simulink model "Pedal_Interpretation_exe_gr"  (Simulink 7.0)
settings: Solver=ode4  StartTime=0.0  StopTime=88  FixedStep=0.01  RelTol=1e-3
InitFcn:
  | PedalInterp_para
values from neighbouring files (symbols this model uses):
  ped_min = 5    [PedalInterp_para.m]
  T_max_Brake = 4000    [PedalInterp_para.m]
  TI = 0    [PAS_callback.m]
undefined symbols (not defined in the file or in its folder): fzgbib, m_ab_100pro, m_ab_70pro, PedalInterpretation, v_bereich
libraries: simulink x320
(part 6 of 23)

== system Pedal_Interpretation_exe_gr/Test Specification for PI/SR-PI-02.1 Brake pedal interpretation/true/PS ==
  A TI1 : Inport  OutDataType=sfix(16)  OutScaling=2^0
  AND : Logic  Inputs=4  AllPortsSameDT=off  OutDataTypeMode=boolean
  Bus Creator : BusCreator  Inputs=3
  Data Type Conversion : DataTypeConversion  OutDataType=sfix(16)  OutScaling=2^0
  Data Type Conversion1 : DataTypeConversion  OutDataType=sfix(16)  OutScaling=2^0
  Data Type Conversion2 : DataTypeConversion  OutDataType=sfix(16)  OutScaling=2^0
  Max Delay A : Subsystem  TreatAsAtomicUnit=on  mask{Delay=0}
      mask prompts: Delay "Delay (in simulation steps) for the input signal:"
      mask init:
      | %set_param([gcb '/Discrete Transfer Fcn'],'Denominator',['[' num2str([1 zeros(1,str2double(get_param(gcb,'Delay')))]) ']']);
      mask CallbackString:
      | Delay = str2double(get_param(gcb,'Delay'));
      | if Delay < 0
      |     set_param(gcb,'Delay','0');
      |     error('Only non-negative delays are possible (causality).');
      |     set_param([gcb '/Delay'],'Value','0');
      | elseif Delay == 0
      |     set_param([gcb '/Delay'],'Value','0');
      | else
      |     set_param([gcb '/Integer Delay'],'NumDelays',num2str(Delay));
      |     set_param([gcb '/Delay'],'Value',num2str(Delay));
      | end
      mask Display: text(0.5,0.5,['z^{ ' num2str((-1)*str2double(get_param(gcb,'Delay'))) '}'],'texmode','on');
  Max Delay R : Subsystem  TreatAsAtomicUnit=on  mask{Delay=0}
      mask prompts: Delay "Delay (in simulation steps) for the input signal:"
      mask init:
      | %set_param([gcb '/Discrete Transfer Fcn'],'Denominator',['[' num2str([1 zeros(1,str2double(get_param(gcb,'Delay')))]) ']']);
      mask CallbackString:
      | Delay = str2double(get_param(gcb,'Delay'));
      | if Delay < 0
      |     set_param(gcb,'Delay','0');
      |     error('Only non-negative delays are possible (causality).');
      |     set_param([gcb '/Delay'],'Value','0');
      | elseif Delay == 0
      |     set_param([gcb '/Delay'],'Value','0');
      | else
      |     set_param([gcb '/Integer Delay'],'NumDelays',num2str(Delay));
      |     set_param([gcb '/Delay'],'Value',num2str(Delay));
      | end
      mask Display: text(0.5,0.5,['z^{ ' num2str((-1)*str2double(get_param(gcb,'Delay'))) '}'],'texmode','on');
  Max Delay T : Subsystem  TreatAsAtomicUnit=on  mask{Delay=0}
      mask prompts: Delay "Delay (in simulation steps) for the input signal:"
      mask init:
      | %set_param([gcb '/Discrete Transfer Fcn'],'Denominator',['[' num2str([1 zeros(1,str2double(get_param(gcb,'Delay')))]) ']']);
      mask CallbackString:
      | Delay = str2double(get_param(gcb,'Delay'));
      | if Delay < 0
      |     set_param(gcb,'Delay','0');
      |     error('Only non-negative delays are possible (causality).');
      |     set_param([gcb '/Delay'],'Value','0');
      | elseif Delay == 0
      |     set_param([gcb '/Delay'],'Value','0');
      | else
      |     set_param([gcb '/Integer Delay'],'NumDelays',num2str(Delay));
      |     set_param([gcb '/Delay'],'Value',num2str(Delay));
      | end
      mask Display: text(0.5,0.5,['z^{ ' num2str((-1)*str2double(get_param(gcb,'Delay'))) '}'],'texmode','on');
  OR - AND : Subsystem
  TDD : Subsystem
  TI : Subsystem
  TID : Subsystem
  Precond : Outport  OutDataType=sfix(16)  OutScaling=2^0
  wires:
  TDD/2(T) -> AND/4
  TID/2(T) -> Max Delay T/1(In1)
  TID/1(A) -> Max Delay A/1(In1)
  Bus Creator/1 -> Precond/1
  Data Type Conversion/1 -> Bus Creator/1  "A"
  Data Type Conversion1/1 -> Bus Creator/2  "T"
  TDD/1(A) -> AND/3
  Max Delay T/1(Out1) -> Data Type Conversion1/1
  Max Delay R/1(Out1) -> AND/1
  Max Delay A/1(Out1) -> Data Type Conversion/1
  AND/1 -> Data Type Conversion2/1
  OR - AND/2(AND) -> TID/2(R AND), Max Delay R/1(In1)
  OR - AND/1(OR) -> TID/1(R OR)
  TI/1(A) -> AND/2
  Data Type Conversion2/1 -> Bus Creator/3  "R"
  A TI1/1 -> TI/1(A1)

== system Pedal_Interpretation_exe_gr/Test Specification for PI/SR-PI-02.2 Acceleration pedal interpretation/T_des_Drive = const/Detect constant ==
  Signal : Inport  OutDataType=sfix(16)  OutScaling=2^0
  Clock : Clock
      settings: Decimation=10
  Constant1 : Constant  Value=0  OutDataTypeMode=boolean  OutDataType=sfix(16)  OutScaling=2^0
  Memory : Memory
  Relative tolerance : Subsystem
  Switch : Switch  Criteria=u2 > Threshold
  Constant : Outport  OutDataType=sfix(16)  OutScaling=2^0
  wires:
  Signal/1 -> Memory/1, Relative tolerance/1(sig)
  Memory/1 -> Relative tolerance/2(ref)
  Constant1/1 -> Switch/3
  Clock/1 -> Switch/2
  Relative tolerance/1(sig == ref) -> Switch/1
  Switch/1 -> Constant/1

== system Pedal_Interpretation_exe_gr/Test Specification for PI/SR-PI-02.2 Acceleration pedal interpretation/T_des_Drive = const/PAS ==
  Precond : Inport  OutDataType=sfix(16)  OutScaling=2^0
  V : Inport  Port=2  OutDataType=sfix(16)  OutScaling=2^0
  A delay : Subsystem  TreatAsAtomicUnit=on  mask{Delay=0}
      mask prompts: Delay "Delay (in simulation steps) for the input signal:"
      mask init:
      | %set_param([gcb '/Discrete Transfer Fcn'],'Denominator',['[' num2str([1 zeros(1,str2double(get_param(gcb,'Delay')))]) ']']);
      mask CallbackString:
      | Delay = str2double(get_param(gcb,'Delay'));
      | if Delay < 0
      |     set_param(gcb,'Delay','0');
      |     error('Only non-negative delays are possible (causality).');
      |     set_param([gcb '/Delay'],'Value','0');
      | elseif Delay == 0
      |     set_param([gcb '/Delay'],'Value','0');
      | else
      |     set_param([gcb '/Integer Delay'],'NumDelays',num2str(Delay));
      |     set_param([gcb '/Delay'],'Value',num2str(Delay));
      | end
      mask Display: text(0.5,0.5,['z^{ ' num2str((-1)*str2double(get_param(gcb,'Delay'))) '}'],'texmode','on');
  AND1 : Logic  AllPortsSameDT=off  OutDataTypeMode=boolean
  Bus Selector : BusSelector  OutputSignals=Local verdict
  Bus Selector1 : BusSelector  OutputSignals=Expected lower limit,Expected upper limit,Actual data
  Bus Selector2 : BusSelector  OutputSignals=R,T,A
  Bus Assignment : BusAssignment  AssignedSignals=Local verdict,Delay
  Bus Assignment1 : BusAssignment  AssignedSignals=Expected lower limit,Expected upper limit,Actual data
  Constant : Constant  Value=-1  OutDataType=sfix(16)  OutScaling=2^0
  Delay bus signals : Subsystem
  Ra delay : Subsystem  TreatAsAtomicUnit=on  mask{Delay=0}
      mask prompts: Delay "Delay (in simulation steps) for the input signal:"
      mask init:
      | %set_param([gcb '/Discrete Transfer Fcn'],'Denominator',['[' num2str([1 zeros(1,str2double(get_param(gcb,'Delay')))]) ']']);
      mask CallbackString:
      | Delay = str2double(get_param(gcb,'Delay'));
      | if Delay < 0
      |     set_param(gcb,'Delay','0');
      |     error('Only non-negative delays are possible (causality).');
      |     set_param([gcb '/Delay'],'Value','0');
      | elseif Delay == 0
      |     set_param([gcb '/Delay'],'Value','0');
      | else
      |     set_param([gcb '/Integer Delay'],'NumDelays',num2str(Delay));
      |     set_param([gcb '/Delay'],'Value',num2str(Delay));
      | end
      mask Display: text(0.5,0.5,['z^{ ' num2str((-1)*str2double(get_param(gcb,'Delay'))) '}'],'texmode','on');
  Rp delay : Subsystem  TreatAsAtomicUnit=on  mask{Delay=0}
      mask prompts: Delay "Delay (in simulation steps) for the input signal:"
      mask init:
      | %set_param([gcb '/Discrete Transfer Fcn'],'Denominator',['[' num2str([1 zeros(1,str2double(get_param(gcb,'Delay')))]) ']']);
      mask CallbackString:
      | Delay = str2double(get_param(gcb,'Delay'));
      | if Delay < 0
      |     set_param(gcb,'Delay','0');
      |     error('Only non-negative delays are possible (causality).');
      |     set_param([gcb '/Delay'],'Value','0');
      | elseif Delay == 0
      |     set_param([gcb '/Delay'],'Value','0');
      | else
      |     set_param([gcb '/Integer Delay'],'NumDelays',num2str(Delay));
      |     set_param([gcb '/Delay'],'Value',num2str(Delay));
      | end
      mask Display: text(0.5,0.5,['z^{ ' num2str((-1)*str2double(get_param(gcb,'Delay'))) '}'],'texmode','on');
  Ta delay : Subsystem  TreatAsAtomicUnit=on  mask{Delay=0}
      mask prompts: Delay "Delay (in simulation steps) for the input signal:"
      mask init:
      | %set_param([gcb '/Discrete Transfer Fcn'],'Denominator',['[' num2str([1 zeros(1,str2double(get_param(gcb,'Delay')))]) ']']);
      mask CallbackString:
      | Delay = str2double(get_param(gcb,'Delay'));
      | if Delay < 0
      |     set_param(gcb,'Delay','0');
      |     error('Only non-negative delays are possible (causality).');
      |     set_param([gcb '/Delay'],'Value','0');
      | elseif Delay == 0
      |     set_param([gcb '/Delay'],'Value','0');
      | else
      |     set_param([gcb '/Integer Delay'],'NumDelays',num2str(Delay));
      |     set_param([gcb '/Delay'],'Value',num2str(Delay));
      | end
      mask Display: text(0.5,0.5,['z^{ ' num2str((-1)*str2double(get_param(gcb,'Delay'))) '}'],'texmode','on');
  Tp delay : Subsystem  TreatAsAtomicUnit=on  mask{Delay=0}
      mask prompts: Delay "Delay (in simulation steps) for the input signal:"
      mask init:
      | %set_param([gcb '/Discrete Transfer Fcn'],'Denominator',['[' num2str([1 zeros(1,str2double(get_param(gcb,'Delay')))]) ']']);
      mask CallbackString:
      | Delay = str2double(get_param(gcb,'Delay'));
      | if Delay < 0
      |     set_param(gcb,'Delay','0');
      |     error('Only non-negative delays are possible (causality).');
      |     set_param([gcb '/Delay'],'Value','0');
      | elseif Delay == 0
      |     set_param([gcb '/Delay'],'Value','0');
      | else
      |     set_param([gcb '/Integer Delay'],'NumDelays',num2str(Delay));
      |     set_param([gcb '/Delay'],'Value',num2str(Delay));
      | end
      mask Display: text(0.5,0.5,['z^{ ' num2str((-1)*str2double(get_param(gcb,'Delay'))) '}'],'texmode','on');
  V delay : Subsystem  TreatAsAtomicUnit=on  mask{Delay=0}
      mask prompts: Delay "Delay (in simulation steps) for the input signal:"
      mask init:
      | %set_param([gcb '/Discrete Transfer Fcn'],'Denominator',['[' num2str([1 zeros(1,str2double(get_param(gcb,'Delay')))]) ']']);
      mask CallbackString:
      | Delay = str2double(get_param(gcb,'Delay'));
      | if Delay < 0
      |     set_param(gcb,'Delay','0');
      |     error('Only non-negative delays are possible (causality).');
      |     set_param([gcb '/Delay'],'Value','0');
      | elseif Delay == 0
      |     set_param([gcb '/Delay'],'Value','0');
      | else
      |     set_param([gcb '/Integer Delay'],'NumDelays',num2str(Delay));
      |     set_param([gcb '/Delay'],'Value',num2str(Delay));
      | end
      mask Display: text(0.5,0.5,['z^{ ' num2str((-1)*str2double(get_param(gcb,'Delay'))) '}'],'texmode','on');
  error : Subsystem
  none - pass - fail : Subsystem
  sw D : Switch  Criteria=u2 ~= 0
  sw V : Switch  Criteria=u2 ~= 0
  VF Info : Outport  OutDataType=sfix(16)  OutScaling=2^0
  wires:
  V/1 -> Bus Selector/1, Bus Selector1/1, Bus Assignment1/1
  error/1(Verror) -> sw V/2, sw D/2
  Constant/1 -> sw V/1
  none - pass - fail/1(Verdict) -> sw V/3
  none - pass - fail/2(MaxDelay) -> sw D/1
  none - pass - fail/3(Delay) -> sw D/3
  sw V/1 -> Bus Assignment/2
  sw D/1 -> Bus Assignment/3
  Bus Selector/1 -> V delay/1(In1), Ra delay/1(In1), Ta delay/1(In1)  "<Local verdict>"
  Bus Assignment/1 -> VF Info/1
  Bus Selector2/1 -> Rp delay/1(In1)  "<R>"
  Bus Selector2/2 -> Tp delay/1(In1)  "<T>"
  Bus Selector2/3 -> A delay/1(In1)  "<A>"
  Rp delay/1(Out1) -> error/1(Rp), none - pass - fail/1(Rp), AND1/1
  Tp delay/1(Out1) -> error/2(Tp), none - pass - fail/2(Tp)
  A delay/1(Out1) -> error/3(A), none - pass - fail/3(A)
  V delay/1(Out1) -> error/6(V), none - pass - fail/6(V)
  Ra delay/1(Out1) -> none - pass - fail/4(Ra), AND1/2, error/4(Ra)
  AND1/1 -> none - pass - fail/7(R AND)
  Precond/1 -> Bus Selector2/1
  Bus Selector1/1 -> Delay bus signals/1(ELLin)  "<Expected lower limit>"
  Bus Selector1/2 -> Delay bus signals/2(EULin)  "<Expected upper limit>"
  Bus Selector1/3 -> Delay bus signals/3(ADin)  "<Actual data>"
  Bus Assignment1/1 -> Bus Assignment/1
  Delay bus signals/1(ELLout) -> Bus Assignment1/2
  Delay bus signals/2(EULout) -> Bus Assignment1/3
  Delay bus signals/3(ADout) -> Bus Assignment1/4
  Ta delay/1(Out1) -> none - pass - fail/5(Ta), error/5(Ta)

== system Pedal_Interpretation_exe_gr/Test Specification for PI/SR-PI-02.2 Acceleration pedal interpretation/T_des_Drive = const/Range - Gap Relative tolerance Ass ==
  Signal : Inport  OutDataType=sfix(16)  OutScaling=2^0
  Reference : Inport  Port=2  OutDataType=sfix(16)  OutScaling=2^0
  Abs : Abs
  Abs1 : Abs
  Add : Sum  Inputs=+-  OutDataType=sfix(16)  OutScaling=2^-10
  Add1 : Sum  Inputs=+-  OutDataType=sfix(16)  OutScaling=2^-10
  Add2 : Sum  OutDataType=sfix(16)  OutScaling=2^-10
  Bus Creator : BusCreator  Inputs=5
  Data Type Conversion : DataTypeConversion  OutDataTypeMode=double  OutDataType=sfix(16)  OutScaling=2^0
  Data Type Conversion1 : DataTypeConversion  OutDataType=sfix(16)  OutScaling=2^0
  Data Type Conversion2 : DataTypeConversion  OutDataType=sfix(16)  OutScaling=2^0
  Data Type Conversion3 : DataTypeConversion  OutDataType=sfix(16)  OutScaling=2^0
  Delay : Constant  Value=0  OutDataType=sfix(16)  OutScaling=2^0
  Divide1 : Product  Inputs=**/  OutDataType=sfix(16)  OutScaling=2^-10
  Max : Constant  Value=100  OutDataType=sfix(16)  OutScaling=2^0
  Relational Operator : RelationalOperator  Operator=<=  LogicOutDataTypeMode=boolean
  Relative Tolerance : Constant  OutDataType=sfix(16)  OutScaling=2^0
  V : Outport  OutDataType=sfix(16)  OutScaling=2^0  InitialOutput=[2]
  wires:
  Data Type Conversion3/1 -> Bus Creator/4  "Actual data"
  Data Type Conversion2/1 -> Bus Creator/3  "Expected upper limit"
  Data Type Conversion1/1 -> Bus Creator/2  "Expected lower limit"
  Data Type Conversion/1 -> Bus Creator/1  "Local verdict"
  Bus Creator/1 -> V/1
  Add1/1 -> Data Type Conversion1/1
  Add2/1 -> Data Type Conversion2/1
  Delay/1 -> Bus Creator/5  "Delay"
  Abs1/1 -> Divide1/1
  Relational Operator/1 -> Data Type Conversion/1
  Relative Tolerance/1 -> Divide1/2
  Max/1 -> Divide1/3
  Divide1/1 -> Add2/1, Add1/2, Relational Operator/2
  Reference/1 -> Add1/1, Add2/2, Abs1/1, Add/2
  Signal/1 -> Data Type Conversion3/1, Add/1
  Add/1 -> Abs/1
  Abs/1 -> Relational Operator/1

== system Pedal_Interpretation_exe_gr/Test Specification for PI/SR-PI-02.2 Acceleration pedal interpretation/T_des_Drive decreases/Detect decrease ==
  Signal : Inport  OutDataType=sfix(16)  OutScaling=2^0
  Clock : Clock
      settings: Decimation=10
  Memory : Memory
  Relational Operator : RelationalOperator  Operator=<  LogicOutDataTypeMode=Specify via dialog
  Switch : Switch  Criteria=u2 > Threshold
  Decrease : Outport  OutDataType=sfix(16)  OutScaling=2^0
  wires:
  Switch/1 -> Relational Operator/2
  Memory/1 -> Switch/1
  Clock/1 -> Switch/2
  Relational Operator/1 -> Decrease/1
  Signal/1 -> Switch/3, Memory/1, Relational Operator/1

== system Pedal_Interpretation_exe_gr/Test Specification for PI/SR-PI-02.2 Acceleration pedal interpretation/T_des_Drive decreases/PAS ==
  Precond : Inport  OutDataType=sfix(16)  OutScaling=2^0
  V : Inport  Port=2  OutDataType=sfix(16)  OutScaling=2^0
  A delay : Subsystem  TreatAsAtomicUnit=on  mask{Delay=0}
      mask prompts: Delay "Delay (in simulation steps) for the input signal:"
      mask init:
      | %set_param([gcb '/Discrete Transfer Fcn'],'Denominator',['[' num2str([1 zeros(1,str2double(get_param(gcb,'Delay')))]) ']']);
      mask CallbackString:
      | Delay = str2double(get_param(gcb,'Delay'));
      | if Delay < 0
      |     set_param(gcb,'Delay','0');
      |     error('Only non-negative delays are possible (causality).');
      |     set_param([gcb '/Delay'],'Value','0');
      | elseif Delay == 0
      |     set_param([gcb '/Delay'],'Value','0');
      | else
      |     set_param([gcb '/Integer Delay'],'NumDelays',num2str(Delay));
      |     set_param([gcb '/Delay'],'Value',num2str(Delay));
      | end
      mask Display: text(0.5,0.5,['z^{ ' num2str((-1)*str2double(get_param(gcb,'Delay'))) '}'],'texmode','on');
  AND1 : Logic  AllPortsSameDT=off  OutDataTypeMode=boolean
  Bus Selector : BusSelector  OutputSignals=Local verdict
  Bus Selector1 : BusSelector  OutputSignals=Expected lower limit,Expected upper limit,Actual data
  Bus Selector2 : BusSelector  OutputSignals=R,T,A
  Bus Assignment : BusAssignment  AssignedSignals=Local verdict,Delay
  Bus Assignment1 : BusAssignment  AssignedSignals=Expected lower limit,Expected upper limit,Actual data
  Constant : Constant  Value=-1  OutDataType=sfix(16)  OutScaling=2^0
  Delay bus signals : Subsystem
  Ra delay : Subsystem  TreatAsAtomicUnit=on  mask{Delay=0}
      mask prompts: Delay "Delay (in simulation steps) for the input signal:"
      mask init:
      | %set_param([gcb '/Discrete Transfer Fcn'],'Denominator',['[' num2str([1 zeros(1,str2double(get_param(gcb,'Delay')))]) ']']);
      mask CallbackString:
      | Delay = str2double(get_param(gcb,'Delay'));
      | if Delay < 0
      |     set_param(gcb,'Delay','0');
      |     error('Only non-negative delays are possible (causality).');
      |     set_param([gcb '/Delay'],'Value','0');
      | elseif Delay == 0
      |     set_param([gcb '/Delay'],'Value','0');
      | else
      |     set_param([gcb '/Integer Delay'],'NumDelays',num2str(Delay));
      |     set_param([gcb '/Delay'],'Value',num2str(Delay));
      | end
      mask Display: text(0.5,0.5,['z^{ ' num2str((-1)*str2double(get_param(gcb,'Delay'))) '}'],'texmode','on');
  Rp delay : Subsystem  TreatAsAtomicUnit=on  mask{Delay=0}
      mask prompts: Delay "Delay (in simulation steps) for the input signal:"
      mask init:
      | %set_param([gcb '/Discrete Transfer Fcn'],'Denominator',['[' num2str([1 zeros(1,str2double(get_param(gcb,'Delay')))]) ']']);
      mask CallbackString:
      | Delay = str2double(get_param(gcb,'Delay'));
      | if Delay < 0
      |     set_param(gcb,'Delay','0');
      |     error('Only non-negative delays are possible (causality).');
      |     set_param([gcb '/Delay'],'Value','0');
      | elseif Delay == 0
      |     set_param([gcb '/Delay'],'Value','0');
      | else
      |     set_param([gcb '/Integer Delay'],'NumDelays',num2str(Delay));
      |     set_param([gcb '/Delay'],'Value',num2str(Delay));
      | end
      mask Display: text(0.5,0.5,['z^{ ' num2str((-1)*str2double(get_param(gcb,'Delay'))) '}'],'texmode','on');
  Ta delay : Subsystem  TreatAsAtomicUnit=on  mask{Delay=0}
      mask prompts: Delay "Delay (in simulation steps) for the input signal:"
      mask init:
      | %set_param([gcb '/Discrete Transfer Fcn'],'Denominator',['[' num2str([1 zeros(1,str2double(get_param(gcb,'Delay')))]) ']']);
      mask CallbackString:
      | Delay = str2double(get_param(gcb,'Delay'));
      | if Delay < 0
      |     set_param(gcb,'Delay','0');
      |     error('Only non-negative delays are possible (causality).');
      |     set_param([gcb '/Delay'],'Value','0');
      | elseif Delay == 0
      |     set_param([gcb '/Delay'],'Value','0');
      | else
      |     set_param([gcb '/Integer Delay'],'NumDelays',num2str(Delay));
      |     set_param([gcb '/Delay'],'Value',num2str(Delay));
      | end
      mask Display: text(0.5,0.5,['z^{ ' num2str((-1)*str2double(get_param(gcb,'Delay'))) '}'],'texmode','on');
  Tp delay : Subsystem  TreatAsAtomicUnit=on  mask{Delay=0}
      mask prompts: Delay "Delay (in simulation steps) for the input signal:"
      mask init:
      | %set_param([gcb '/Discrete Transfer Fcn'],'Denominator',['[' num2str([1 zeros(1,str2double(get_param(gcb,'Delay')))]) ']']);
      mask CallbackString:
      | Delay = str2double(get_param(gcb,'Delay'));
      | if Delay < 0
      |     set_param(gcb,'Delay','0');
      |     error('Only non-negative delays are possible (causality).');
      |     set_param([gcb '/Delay'],'Value','0');
      | elseif Delay == 0
      |     set_param([gcb '/Delay'],'Value','0');
      | else
      |     set_param([gcb '/Integer Delay'],'NumDelays',num2str(Delay));
      |     set_param([gcb '/Delay'],'Value',num2str(Delay));
      | end
      mask Display: text(0.5,0.5,['z^{ ' num2str((-1)*str2double(get_param(gcb,'Delay'))) '}'],'texmode','on');
  V delay : Subsystem  TreatAsAtomicUnit=on  mask{Delay=0}
      mask prompts: Delay "Delay (in simulation steps) for the input signal:"
      mask init:
      | %set_param([gcb '/Discrete Transfer Fcn'],'Denominator',['[' num2str([1 zeros(1,str2double(get_param(gcb,'Delay')))]) ']']);
      mask CallbackString:
      | Delay = str2double(get_param(gcb,'Delay'));
      | if Delay < 0
      |     set_param(gcb,'Delay','0');
      |     error('Only non-negative delays are possible (causality).');
      |     set_param([gcb '/Delay'],'Value','0');
      | elseif Delay == 0
      |     set_param([gcb '/Delay'],'Value','0');
      | else
      |     set_param([gcb '/Integer Delay'],'NumDelays',num2str(Delay));
      |     set_param([gcb '/Delay'],'Value',num2str(Delay));
      | end
      mask Display: text(0.5,0.5,['z^{ ' num2str((-1)*str2double(get_param(gcb,'Delay'))) '}'],'texmode','on');
  error : Subsystem
  none - pass - fail : Subsystem
  sw D : Switch  Criteria=u2 ~= 0
  sw V : Switch  Criteria=u2 ~= 0
  VF Info : Outport  OutDataType=sfix(16)  OutScaling=2^0
  wires:
  V/1 -> Bus Selector/1, Bus Selector1/1, Bus Assignment1/1
  error/1(Verror) -> sw V/2, sw D/2
  Constant/1 -> sw V/1
  none - pass - fail/1(Verdict) -> sw V/3
  none - pass - fail/2(MaxDelay) -> sw D/1
  none - pass - fail/3(Delay) -> sw D/3
  sw V/1 -> Bus Assignment/2
  sw D/1 -> Bus Assignment/3
  Bus Selector/1 -> V delay/1(In1), Ra delay/1(In1), Ta delay/1(In1)  "<Local verdict>"
  Bus Assignment/1 -> VF Info/1
  Bus Selector2/1 -> Rp delay/1(In1)  "<R>"
  Bus Selector2/2 -> Tp delay/1(In1)  "<T>"
  Bus Selector2/3 -> A delay/1(In1)  "<A>"
  Rp delay/1(Out1) -> error/1(Rp), none - pass - fail/1(Rp), AND1/1
  Tp delay/1(Out1) -> error/2(Tp), none - pass - fail/2(Tp)
  A delay/1(Out1) -> error/3(A), none - pass - fail/3(A)
  V delay/1(Out1) -> error/6(V), none - pass - fail/6(V)
  Ra delay/1(Out1) -> none - pass - fail/4(Ra), AND1/2, error/4(Ra)
  AND1/1 -> none - pass - fail/7(R AND)
  Precond/1 -> Bus Selector2/1
  Bus Selector1/1 -> Delay bus signals/1(ELLin)  "<Expected lower limit>"
  Bus Selector1/2 -> Delay bus signals/2(EULin)  "<Expected upper limit>"
  Bus Selector1/3 -> Delay bus signals/3(ADin)  "<Actual data>"
  Bus Assignment1/1 -> Bus Assignment/1
  Delay bus signals/1(ELLout) -> Bus Assignment1/2
  Delay bus signals/2(EULout) -> Bus Assignment1/3
  Delay bus signals/3(ADout) -> Bus Assignment1/4
  Ta delay/1(Out1) -> none - pass - fail/5(Ta), error/5(Ta)

== system Pedal_Interpretation_exe_gr/Test Specification for PI/SR-PI-02.2 Acceleration pedal interpretation/T_des_Drive decreases/Range - Gap Relative tolerance Ass ==
  Signal : Inport  OutDataType=sfix(16)  OutScaling=2^0
  Reference : Inport  Port=2  OutDataType=sfix(16)  OutScaling=2^0
  Abs : Abs
  Abs1 : Abs
  Add : Sum  Inputs=+-  OutDataType=sfix(16)  OutScaling=2^-10
  Add1 : Sum  Inputs=+-  OutDataType=sfix(16)  OutScaling=2^-10
  Add2 : Sum  OutDataType=sfix(16)  OutScaling=2^-10
  Bus Creator : BusCreator  Inputs=5
  Data Type Conversion : DataTypeConversion  OutDataTypeMode=double  OutDataType=sfix(16)  OutScaling=2^0
  Data Type Conversion1 : DataTypeConversion  OutDataType=sfix(16)  OutScaling=2^0
  Data Type Conversion2 : DataTypeConversion  OutDataType=sfix(16)  OutScaling=2^0
  Data Type Conversion3 : DataTypeConversion  OutDataType=sfix(16)  OutScaling=2^0
  Delay : Constant  Value=0  OutDataType=sfix(16)  OutScaling=2^0
  Divide1 : Product  Inputs=**/  OutDataType=sfix(16)  OutScaling=2^-10
  Max : Constant  Value=100  OutDataType=sfix(16)  OutScaling=2^0
  Relational Operator : RelationalOperator  Operator=<=  LogicOutDataTypeMode=boolean
  Relative Tolerance : Constant  OutDataType=sfix(16)  OutScaling=2^0
  V : Outport  OutDataType=sfix(16)  OutScaling=2^0  InitialOutput=[2]
  wires:
  Data Type Conversion3/1 -> Bus Creator/4  "Actual data"
  Data Type Conversion2/1 -> Bus Creator/3  "Expected upper limit"
  Data Type Conversion1/1 -> Bus Creator/2  "Expected lower limit"
  Data Type Conversion/1 -> Bus Creator/1  "Local verdict"
  Bus Creator/1 -> V/1
  Add1/1 -> Data Type Conversion1/1
  Add2/1 -> Data Type Conversion2/1
  Delay/1 -> Bus Creator/5  "Delay"
  Abs1/1 -> Divide1/1
  Relational Operator/1 -> Data Type Conversion/1
  Relative Tolerance/1 -> Divide1/2
  Max/1 -> Divide1/3
  Divide1/1 -> Add2/1, Add1/2, Relational Operator/2
  Reference/1 -> Add1/1, Add2/2, Abs1/1, Add/2
  Signal/1 -> Data Type Conversion3/1, Add/1
  Add/1 -> Abs/1
  Abs/1 -> Relational Operator/1

== system Pedal_Interpretation_exe_gr/Test Specification for PI/SR-PI-02.2 Acceleration pedal interpretation/T_des_Drive decreases /Detect decrease ==
  Signal : Inport  OutDataType=sfix(16)  OutScaling=2^0
  Clock : Clock
      settings: Decimation=10
  Memory : Memory
  Relational Operator : RelationalOperator  Operator=<  LogicOutDataTypeMode=Specify via dialog
  Switch : Switch  Criteria=u2 > Threshold
  Decrease : Outport  OutDataType=sfix(16)  OutScaling=2^0
  wires:
  Switch/1 -> Relational Operator/2
  Memory/1 -> Switch/1
  Clock/1 -> Switch/2
  Relational Operator/1 -> Decrease/1
  Signal/1 -> Switch/3, Memory/1, Relational Operator/1

== system Pedal_Interpretation_exe_gr/Test Specification for PI/SR-PI-02.2 Acceleration pedal interpretation/T_des_Drive decreases /PAS ==
  Precond : Inport  OutDataType=sfix(16)  OutScaling=2^0
  V : Inport  Port=2  OutDataType=sfix(16)  OutScaling=2^0
  A delay : Subsystem  TreatAsAtomicUnit=on  mask{Delay=0}
      mask prompts: Delay "Delay (in simulation steps) for the input signal:"
      mask init:
      | %set_param([gcb '/Discrete Transfer Fcn'],'Denominator',['[' num2str([1 zeros(1,str2double(get_param(gcb,'Delay')))]) ']']);
      mask CallbackString:
      | Delay = str2double(get_param(gcb,'Delay'));
      | if Delay < 0
      |     set_param(gcb,'Delay','0');
      |     error('Only non-negative delays are possible (causality).');
      |     set_param([gcb '/Delay'],'Value','0');
      | elseif Delay == 0
      |     set_param([gcb '/Delay'],'Value','0');
      | else
      |     set_param([gcb '/Integer Delay'],'NumDelays',num2str(Delay));
      |     set_param([gcb '/Delay'],'Value',num2str(Delay));
      | end
      mask Display: text(0.5,0.5,['z^{ ' num2str((-1)*str2double(get_param(gcb,'Delay'))) '}'],'texmode','on');
  AND1 : Logic  AllPortsSameDT=off  OutDataTypeMode=boolean
  Bus Selector : BusSelector  OutputSignals=Local verdict
  Bus Selector1 : BusSelector  OutputSignals=Expected lower limit,Expected upper limit,Actual data
  Bus Selector2 : BusSelector  OutputSignals=R,T,A
  Bus Assignment : BusAssignment  AssignedSignals=Local verdict,Delay
  Bus Assignment1 : BusAssignment  AssignedSignals=Expected lower limit,Expected upper limit,Actual data
  Constant : Constant  Value=-1  OutDataType=sfix(16)  OutScaling=2^0
  Delay bus signals : Subsystem
  Ra delay : Subsystem  TreatAsAtomicUnit=on  mask{Delay=0}
      mask prompts: Delay "Delay (in simulation steps) for the input signal:"
      mask init:
      | %set_param([gcb '/Discrete Transfer Fcn'],'Denominator',['[' num2str([1 zeros(1,str2double(get_param(gcb,'Delay')))]) ']']);
      mask CallbackString:
      | Delay = str2double(get_param(gcb,'Delay'));
      | if Delay < 0
      |     set_param(gcb,'Delay','0');
      |     error('Only non-negative delays are possible (causality).');
      |     set_param([gcb '/Delay'],'Value','0');
      | elseif Delay == 0
      |     set_param([gcb '/Delay'],'Value','0');
      | else
      |     set_param([gcb '/Integer Delay'],'NumDelays',num2str(Delay));
      |     set_param([gcb '/Delay'],'Value',num2str(Delay));
      | end
      mask Display: text(0.5,0.5,['z^{ ' num2str((-1)*str2double(get_param(gcb,'Delay'))) '}'],'texmode','on');
  Rp delay : Subsystem  TreatAsAtomicUnit=on  mask{Delay=0}
      mask prompts: Delay "Delay (in simulation steps) for the input signal:"
      mask init:
      | %set_param([gcb '/Discrete Transfer Fcn'],'Denominator',['[' num2str([1 zeros(1,str2double(get_param(gcb,'Delay')))]) ']']);
      mask CallbackString:
      | Delay = str2double(get_param(gcb,'Delay'));
      | if Delay < 0
      |     set_param(gcb,'Delay','0');
      |     error('Only non-negative delays are possible (causality).');
      |     set_param([gcb '/Delay'],'Value','0');
      | elseif Delay == 0
      |     set_param([gcb '/Delay'],'Value','0');
      | else
      |     set_param([gcb '/Integer Delay'],'NumDelays',num2str(Delay));
      |     set_param([gcb '/Delay'],'Value',num2str(Delay));
      | end
      mask Display: text(0.5,0.5,['z^{ ' num2str((-1)*str2double(get_param(gcb,'Delay'))) '}'],'texmode','on');
  Ta delay : Subsystem  TreatAsAtomicUnit=on  mask{Delay=0}
      mask prompts: Delay "Delay (in simulation steps) for the input signal:"
      mask init:
      | %set_param([gcb '/Discrete Transfer Fcn'],'Denominator',['[' num2str([1 zeros(1,str2double(get_param(gcb,'Delay')))]) ']']);
      mask CallbackString:
      | Delay = str2double(get_param(gcb,'Delay'));
      | if Delay < 0
      |     set_param(gcb,'Delay','0');
      |     error('Only non-negative delays are possible (causality).');
      |     set_param([gcb '/Delay'],'Value','0');
      | elseif Delay == 0
      |     set_param([gcb '/Delay'],'Value','0');
      | else
      |     set_param([gcb '/Integer Delay'],'NumDelays',num2str(Delay));
      |     set_param([gcb '/Delay'],'Value',num2str(Delay));
      | end
      mask Display: text(0.5,0.5,['z^{ ' num2str((-1)*str2double(get_param(gcb,'Delay'))) '}'],'texmode','on');
  Tp delay : Subsystem  TreatAsAtomicUnit=on  mask{Delay=0}
      mask prompts: Delay "Delay (in simulation steps) for the input signal:"
      mask init:
      | %set_param([gcb '/Discrete Transfer Fcn'],'Denominator',['[' num2str([1 zeros(1,str2double(get_param(gcb,'Delay')))]) ']']);
      mask CallbackString:
      | Delay = str2double(get_param(gcb,'Delay'));
      | if Delay < 0
      |     set_param(gcb,'Delay','0');
      |     error('Only non-negative delays are possible (causality).');
      |     set_param([gcb '/Delay'],'Value','0');
      | elseif Delay == 0
      |     set_param([gcb '/Delay'],'Value','0');
      | else
      |     set_param([gcb '/Integer Delay'],'NumDelays',num2str(Delay));
      |     set_param([gcb '/Delay'],'Value',num2str(Delay));
      | end
      mask Display: text(0.5,0.5,['z^{ ' num2str((-1)*str2double(get_param(gcb,'Delay'))) '}'],'texmode','on');
  V delay : Subsystem  TreatAsAtomicUnit=on  mask{Delay=0}
      mask prompts: Delay "Delay (in simulation steps) for the input signal:"
      mask init:
      | %set_param([gcb '/Discrete Transfer Fcn'],'Denominator',['[' num2str([1 zeros(1,str2double(get_param(gcb,'Delay')))]) ']']);
      mask CallbackString:
      | Delay = str2double(get_param(gcb,'Delay'));
      | if Delay < 0
      |     set_param(gcb,'Delay','0');
      |     error('Only non-negative delays are possible (causality).');
      |     set_param([gcb '/Delay'],'Value','0');
      | elseif Delay == 0
      |     set_param([gcb '/Delay'],'Value','0');
      | else
      |     set_param([gcb '/Integer Delay'],'NumDelays',num2str(Delay));
      |     set_param([gcb '/Delay'],'Value',num2str(Delay));
      | end
      mask Display: text(0.5,0.5,['z^{ ' num2str((-1)*str2double(get_param(gcb,'Delay'))) '}'],'texmode','on');
  error : Subsystem
  none - pass - fail : Subsystem
  sw D : Switch  Criteria=u2 ~= 0
  sw V : Switch  Criteria=u2 ~= 0
  VF Info : Outport  OutDataType=sfix(16)  OutScaling=2^0
  wires:
  V/1 -> Bus Selector/1, Bus Selector1/1, Bus Assignment1/1
  error/1(Verror) -> sw V/2, sw D/2
  Constant/1 -> sw V/1
  none - pass - fail/1(Verdict) -> sw V/3
  none - pass - fail/2(MaxDelay) -> sw D/1
  none - pass - fail/3(Delay) -> sw D/3
  sw V/1 -> Bus Assignment/2
  sw D/1 -> Bus Assignment/3
  Bus Selector/1 -> V delay/1(In1), Ra delay/1(In1), Ta delay/1(In1)  "<Local verdict>"
  Bus Assignment/1 -> VF Info/1
  Bus Selector2/1 -> Rp delay/1(In1)  "<R>"
  Bus Selector2/2 -> Tp delay/1(In1)  "<T>"
  Bus Selector2/3 -> A delay/1(In1)  "<A>"
  Rp delay/1(Out1) -> error/1(Rp), none - pass - fail/1(Rp), AND1/1
  Tp delay/1(Out1) -> error/2(Tp), none - pass - fail/2(Tp)
  A delay/1(Out1) -> error/3(A), none - pass - fail/3(A)
  V delay/1(Out1) -> error/6(V), none - pass - fail/6(V)
  Ra delay/1(Out1) -> none - pass - fail/4(Ra), AND1/2, error/4(Ra)
  AND1/1 -> none - pass - fail/7(R AND)
  Precond/1 -> Bus Selector2/1
  Bus Selector1/1 -> Delay bus signals/1(ELLin)  "<Expected lower limit>"
  Bus Selector1/2 -> Delay bus signals/2(EULin)  "<Expected upper limit>"
  Bus Selector1/3 -> Delay bus signals/3(ADin)  "<Actual data>"
  Bus Assignment1/1 -> Bus Assignment/1
  Delay bus signals/1(ELLout) -> Bus Assignment1/2
  Delay bus signals/2(EULout) -> Bus Assignment1/3
  Delay bus signals/3(ADout) -> Bus Assignment1/4
  Ta delay/1(Out1) -> none - pass - fail/5(Ta), error/5(Ta)

== system Pedal_Interpretation_exe_gr/Test Specification for PI/SR-PI-02.2 Acceleration pedal interpretation/T_des_Drive decreases /Range - Gap Relative tolerance Ass ==
  Signal : Inport  OutDataType=sfix(16)  OutScaling=2^0
  Reference : Inport  Port=2  OutDataType=sfix(16)  OutScaling=2^0
  Abs : Abs
  Abs1 : Abs
  Add : Sum  Inputs=+-  OutDataType=sfix(16)  OutScaling=2^-10
  Add1 : Sum  Inputs=+-  OutDataType=sfix(16)  OutScaling=2^-10
  Add2 : Sum  OutDataType=sfix(16)  OutScaling=2^-10
  Bus Creator : BusCreator  Inputs=5
  Data Type Conversion : DataTypeConversion  OutDataTypeMode=double  OutDataType=sfix(16)  OutScaling=2^0
  Data Type Conversion1 : DataTypeConversion  OutDataType=sfix(16)  OutScaling=2^0
  Data Type Conversion2 : DataTypeConversion  OutDataType=sfix(16)  OutScaling=2^0
  Data Type Conversion3 : DataTypeConversion  OutDataType=sfix(16)  OutScaling=2^0
  Delay : Constant  Value=0  OutDataType=sfix(16)  OutScaling=2^0
  Divide1 : Product  Inputs=**/  OutDataType=sfix(16)  OutScaling=2^-10
  Max : Constant  Value=100  OutDataType=sfix(16)  OutScaling=2^0
  Relational Operator : RelationalOperator  Operator=<=  LogicOutDataTypeMode=boolean
  Relative Tolerance : Constant  OutDataType=sfix(16)  OutScaling=2^0
  V : Outport  OutDataType=sfix(16)  OutScaling=2^0  InitialOutput=[2]
  wires:
  Data Type Conversion3/1 -> Bus Creator/4  "Actual data"
  Data Type Conversion2/1 -> Bus Creator/3  "Expected upper limit"
  Data Type Conversion1/1 -> Bus Creator/2  "Expected lower limit"
  Data Type Conversion/1 -> Bus Creator/1  "Local verdict"
  Bus Creator/1 -> V/1
  Add1/1 -> Data Type Conversion1/1
  Add2/1 -> Data Type Conversion2/1
  Delay/1 -> Bus Creator/5  "Delay"
  Abs1/1 -> Divide1/1
  Relational Operator/1 -> Data Type Conversion/1
  Relative Tolerance/1 -> Divide1/2
  Max/1 -> Divide1/3
  Divide1/1 -> Add2/1, Add1/2, Relational Operator/2
  Reference/1 -> Add1/1, Add2/2, Abs1/1, Add/2
  Signal/1 -> Data Type Conversion3/1, Add/1
  Add/1 -> Abs/1
  Abs/1 -> Relational Operator/1

== system Pedal_Interpretation_exe_gr/Test Specification for PI/SR-PI-02.2 Acceleration pedal interpretation/T_des_Drive does not increase/Detect 'does not increase' ==
  Signal : Inport  OutDataType=sfix(16)  OutScaling=2^0
  Clock : Clock
      settings: Decimation=10
  Memory : Memory
  Relational Operator : RelationalOperator  Operator=<=  LogicOutDataTypeMode=Specify via dialog
  Switch : Switch  Criteria=u2 > Threshold
  Decrease : Outport  OutDataType=sfix(16)  OutScaling=2^0
  wires:
  Switch/1 -> Relational Operator/2
  Memory/1 -> Switch/1
  Clock/1 -> Switch/2
  Relational Operator/1 -> Decrease/1
  Signal/1 -> Switch/3, Memory/1, Relational Operator/1

== system Pedal_Interpretation_exe_gr/Test Specification for PI/SR-PI-02.2 Acceleration pedal interpretation/T_des_Drive does not increase/PAS ==
  Precond : Inport  OutDataType=sfix(16)  OutScaling=2^0
  V : Inport  Port=2  OutDataType=sfix(16)  OutScaling=2^0
  A delay : Subsystem  TreatAsAtomicUnit=on  mask{Delay=0}
      mask prompts: Delay "Delay (in simulation steps) for the input signal:"
      mask init:
      | %set_param([gcb '/Discrete Transfer Fcn'],'Denominator',['[' num2str([1 zeros(1,str2double(get_param(gcb,'Delay')))]) ']']);
      mask CallbackString:
      | Delay = str2double(get_param(gcb,'Delay'));
      | if Delay < 0
      |     set_param(gcb,'Delay','0');
      |     error('Only non-negative delays are possible (causality).');
      |     set_param([gcb '/Delay'],'Value','0');
      | elseif Delay == 0
      |     set_param([gcb '/Delay'],'Value','0');
      | else
      |     set_param([gcb '/Integer Delay'],'NumDelays',num2str(Delay));
      |     set_param([gcb '/Delay'],'Value',num2str(Delay));
      | end
      mask Display: text(0.5,0.5,['z^{ ' num2str((-1)*str2double(get_param(gcb,'Delay'))) '}'],'texmode','on');
  AND1 : Logic  AllPortsSameDT=off  OutDataTypeMode=boolean
  Bus Selector : BusSelector  OutputSignals=Local verdict
  Bus Selector1 : BusSelector  OutputSignals=Expected lower limit,Expected upper limit,Actual data
  Bus Selector2 : BusSelector  OutputSignals=R,T,A
  Bus Assignment : BusAssignment  AssignedSignals=Local verdict,Delay
  Bus Assignment1 : BusAssignment  AssignedSignals=Expected lower limit,Expected upper limit,Actual data
  Constant : Constant  Value=-1  OutDataType=sfix(16)  OutScaling=2^0
  Delay bus signals : Subsystem
  Ra delay : Subsystem  TreatAsAtomicUnit=on  mask{Delay=0}
      mask prompts: Delay "Delay (in simulation steps) for the input signal:"
      mask init:
      | %set_param([gcb '/Discrete Transfer Fcn'],'Denominator',['[' num2str([1 zeros(1,str2double(get_param(gcb,'Delay')))]) ']']);
      mask CallbackString:
      | Delay = str2double(get_param(gcb,'Delay'));
      | if Delay < 0
      |     set_param(gcb,'Delay','0');
      |     error('Only non-negative delays are possible (causality).');
      |     set_param([gcb '/Delay'],'Value','0');
      | elseif Delay == 0
      |     set_param([gcb '/Delay'],'Value','0');
      | else
      |     set_param([gcb '/Integer Delay'],'NumDelays',num2str(Delay));
      |     set_param([gcb '/Delay'],'Value',num2str(Delay));
      | end
      mask Display: text(0.5,0.5,['z^{ ' num2str((-1)*str2double(get_param(gcb,'Delay'))) '}'],'texmode','on');
  Rp delay : Subsystem  TreatAsAtomicUnit=on  mask{Delay=0}
      mask prompts: Delay "Delay (in simulation steps) for the input signal:"
      mask init:
      | %set_param([gcb '/Discrete Transfer Fcn'],'Denominator',['[' num2str([1 zeros(1,str2double(get_param(gcb,'Delay')))]) ']']);
      mask CallbackString:
      | Delay = str2double(get_param(gcb,'Delay'));
      | if Delay < 0
      |     set_param(gcb,'Delay','0');
      |     error('Only non-negative delays are possible (causality).');
      |     set_param([gcb '/Delay'],'Value','0');
      | elseif Delay == 0
      |     set_param([gcb '/Delay'],'Value','0');
      | else
      |     set_param([gcb '/Integer Delay'],'NumDelays',num2str(Delay));
      |     set_param([gcb '/Delay'],'Value',num2str(Delay));
      | end
      mask Display: text(0.5,0.5,['z^{ ' num2str((-1)*str2double(get_param(gcb,'Delay'))) '}'],'texmode','on');
  Ta delay : Subsystem  TreatAsAtomicUnit=on  mask{Delay=0}
      mask prompts: Delay "Delay (in simulation steps) for the input signal:"
      mask init:
      | %set_param([gcb '/Discrete Transfer Fcn'],'Denominator',['[' num2str([1 zeros(1,str2double(get_param(gcb,'Delay')))]) ']']);
      mask CallbackString:
      | Delay = str2double(get_param(gcb,'Delay'));
      | if Delay < 0
      |     set_param(gcb,'Delay','0');
      |     error('Only non-negative delays are possible (causality).');
      |     set_param([gcb '/Delay'],'Value','0');
      | elseif Delay == 0
      |     set_param([gcb '/Delay'],'Value','0');
      | else
      |     set_param([gcb '/Integer Delay'],'NumDelays',num2str(Delay));
      |     set_param([gcb '/Delay'],'Value',num2str(Delay));
      | end
      mask Display: text(0.5,0.5,['z^{ ' num2str((-1)*str2double(get_param(gcb,'Delay'))) '}'],'texmode','on');
  Tp delay : Subsystem  TreatAsAtomicUnit=on  mask{Delay=0}
      mask prompts: Delay "Delay (in simulation steps) for the input signal:"
      mask init:
      | %set_param([gcb '/Discrete Transfer Fcn'],'Denominator',['[' num2str([1 zeros(1,str2double(get_param(gcb,'Delay')))]) ']']);
      mask CallbackString:
      | Delay = str2double(get_param(gcb,'Delay'));
      | if Delay < 0
      |     set_param(gcb,'Delay','0');
      |     error('Only non-negative delays are possible (causality).');
      |     set_param([gcb '/Delay'],'Value','0');
      | elseif Delay == 0
      |     set_param([gcb '/Delay'],'Value','0');
      | else
      |     set_param([gcb '/Integer Delay'],'NumDelays',num2str(Delay));
      |     set_param([gcb '/Delay'],'Value',num2str(Delay));
      | end
      mask Display: text(0.5,0.5,['z^{ ' num2str((-1)*str2double(get_param(gcb,'Delay'))) '}'],'texmode','on');
  V delay : Subsystem  TreatAsAtomicUnit=on  mask{Delay=0}
      mask prompts: Delay "Delay (in simulation steps) for the input signal:"
      mask init:
      | %set_param([gcb '/Discrete Transfer Fcn'],'Denominator',['[' num2str([1 zeros(1,str2double(get_param(gcb,'Delay')))]) ']']);
      mask CallbackString:
      | Delay = str2double(get_param(gcb,'Delay'));
      | if Delay < 0
      |     set_param(gcb,'Delay','0');
      |     error('Only non-negative delays are possible (causality).');
      |     set_param([gcb '/Delay'],'Value','0');
      | elseif Delay == 0
      |     set_param([gcb '/Delay'],'Value','0');
      | else
      |     set_param([gcb '/Integer Delay'],'NumDelays',num2str(Delay));
      |     set_param([gcb '/Delay'],'Value',num2str(Delay));
      | end
      mask Display: text(0.5,0.5,['z^{ ' num2str((-1)*str2double(get_param(gcb,'Delay'))) '}'],'texmode','on');
  error : Subsystem
  none - pass - fail : Subsystem
  sw D : Switch  Criteria=u2 ~= 0
  sw V : Switch  Criteria=u2 ~= 0
  VF Info : Outport  OutDataType=sfix(16)  OutScaling=2^0
  wires:
  V/1 -> Bus Selector/1, Bus Selector1/1, Bus Assignment1/1
  error/1(Verror) -> sw V/2, sw D/2
  Constant/1 -> sw V/1
  none - pass - fail/1(Verdict) -> sw V/3
  none - pass - fail/2(MaxDelay) -> sw D/1
  none - pass - fail/3(Delay) -> sw D/3
  sw V/1 -> Bus Assignment/2
  sw D/1 -> Bus Assignment/3
  Bus Selector/1 -> V delay/1(In1), Ra delay/1(In1), Ta delay/1(In1)  "<Local verdict>"
  Bus Assignment/1 -> VF Info/1
  Bus Selector2/1 -> Rp delay/1(In1)  "<R>"
  Bus Selector2/2 -> Tp delay/1(In1)  "<T>"
  Bus Selector2/3 -> A delay/1(In1)  "<A>"
  Rp delay/1(Out1) -> error/1(Rp), none - pass - fail/1(Rp), AND1/1
  Tp delay/1(Out1) -> error/2(Tp), none - pass - fail/2(Tp)
  A delay/1(Out1) -> error/3(A), none - pass - fail/3(A)
  V delay/1(Out1) -> error/6(V), none - pass - fail/6(V)
  Ra delay/1(Out1) -> none - pass - fail/4(Ra), AND1/2, error/4(Ra)
  AND1/1 -> none - pass - fail/7(R AND)
  Precond/1 -> Bus Selector2/1
  Bus Selector1/1 -> Delay bus signals/1(ELLin)  "<Expected lower limit>"
  Bus Selector1/2 -> Delay bus signals/2(EULin)  "<Expected upper limit>"
  Bus Selector1/3 -> Delay bus signals/3(ADin)  "<Actual data>"
  Bus Assignment1/1 -> Bus Assignment/1
  Delay bus signals/1(ELLout) -> Bus Assignment1/2
  Delay bus signals/2(EULout) -> Bus Assignment1/3
  Delay bus signals/3(ADout) -> Bus Assignment1/4
  Ta delay/1(Out1) -> none - pass - fail/5(Ta), error/5(Ta)

== system Pedal_Interpretation_exe_gr/Test Specification for PI/SR-PI-02.2 Acceleration pedal interpretation/T_des_Drive does not increase/Range - Gap Relative tolerance Ass ==
  Signal : Inport  OutDataType=sfix(16)  OutScaling=2^0
  Reference : Inport  Port=2  OutDataType=sfix(16)  OutScaling=2^0
  Abs : Abs
  Abs1 : Abs
  Add : Sum  Inputs=+-  OutDataType=sfix(16)  OutScaling=2^-10
  Add1 : Sum  Inputs=+-  OutDataType=sfix(16)  OutScaling=2^-10
  Add2 : Sum  OutDataType=sfix(16)  OutScaling=2^-10
  Bus Creator : BusCreator  Inputs=5
  Data Type Conversion : DataTypeConversion  OutDataTypeMode=double  OutDataType=sfix(16)  OutScaling=2^0
  Data Type Conversion1 : DataTypeConversion  OutDataType=sfix(16)  OutScaling=2^0
  Data Type Conversion2 : DataTypeConversion  OutDataType=sfix(16)  OutScaling=2^0
  Data Type Conversion3 : DataTypeConversion  OutDataType=sfix(16)  OutScaling=2^0
  Delay : Constant  Value=0  OutDataType=sfix(16)  OutScaling=2^0
  Divide1 : Product  Inputs=**/  OutDataType=sfix(16)  OutScaling=2^-10
  Max : Constant  Value=100  OutDataType=sfix(16)  OutScaling=2^0
  Relational Operator : RelationalOperator  Operator=<=  LogicOutDataTypeMode=boolean
  Relative Tolerance : Constant  OutDataType=sfix(16)  OutScaling=2^0
  V : Outport  OutDataType=sfix(16)  OutScaling=2^0  InitialOutput=[2]
  wires:
  Data Type Conversion3/1 -> Bus Creator/4  "Actual data"
  Data Type Conversion2/1 -> Bus Creator/3  "Expected upper limit"
  Data Type Conversion1/1 -> Bus Creator/2  "Expected lower limit"
  Data Type Conversion/1 -> Bus Creator/1  "Local verdict"
  Bus Creator/1 -> V/1
  Add1/1 -> Data Type Conversion1/1
  Add2/1 -> Data Type Conversion2/1
  Delay/1 -> Bus Creator/5  "Delay"
  Abs1/1 -> Divide1/1
  Relational Operator/1 -> Data Type Conversion/1
  Relative Tolerance/1 -> Divide1/2
  Max/1 -> Divide1/3
  Divide1/1 -> Add2/1, Add1/2, Relational Operator/2
  Reference/1 -> Add1/1, Add2/2, Abs1/1, Add/2
  Signal/1 -> Data Type Conversion3/1, Add/1
  Add/1 -> Abs/1
  Abs/1 -> Relational Operator/1

== system Pedal_Interpretation_exe_gr/Test Specification for PI/SR-PI-02.2 Acceleration pedal interpretation/T_des_Drive increases/   ==
  Signal : Inport  OutDataType=sfix(16)  OutScaling=2^0
  Reference : Inport  Port=2  OutDataType=sfix(16)  OutScaling=2^0
  Abs : Abs
  Abs1 : Abs
  Add : Sum  Inputs=+-  OutDataType=sfix(16)  OutScaling=2^-10
  Add1 : Sum  Inputs=+-  OutDataType=sfix(16)  OutScaling=2^-10
  Add2 : Sum  OutDataType=sfix(16)  OutScaling=2^-10
  Bus Creator : BusCreator  Inputs=5
  Data Type Conversion : DataTypeConversion  OutDataTypeMode=double  OutDataType=sfix(16)  OutScaling=2^0
  Data Type Conversion1 : DataTypeConversion  OutDataType=sfix(16)  OutScaling=2^0
  Data Type Conversion2 : DataTypeConversion  OutDataType=sfix(16)  OutScaling=2^0
  Data Type Conversion3 : DataTypeConversion  OutDataType=sfix(16)  OutScaling=2^0
  Delay : Constant  Value=0  OutDataType=sfix(16)  OutScaling=2^0
  Divide1 : Product  Inputs=**/  OutDataType=sfix(16)  OutScaling=2^-10
  Max : Constant  Value=100  OutDataType=sfix(16)  OutScaling=2^0
  Relational Operator : RelationalOperator  Operator=<=  LogicOutDataTypeMode=boolean
  Relative Tolerance : Constant  OutDataType=sfix(16)  OutScaling=2^0
  V : Outport  OutDataType=sfix(16)  OutScaling=2^0  InitialOutput=[2]
  wires:
  Data Type Conversion3/1 -> Bus Creator/4  "Actual data"
  Data Type Conversion2/1 -> Bus Creator/3  "Expected upper limit"
  Data Type Conversion1/1 -> Bus Creator/2  "Expected lower limit"
  Data Type Conversion/1 -> Bus Creator/1  "Local verdict"
  Bus Creator/1 -> V/1
  Add1/1 -> Data Type Conversion1/1
  Add2/1 -> Data Type Conversion2/1
  Delay/1 -> Bus Creator/5  "Delay"
  Abs1/1 -> Divide1/1
  Relational Operator/1 -> Data Type Conversion/1
  Relative Tolerance/1 -> Divide1/2
  Max/1 -> Divide1/3
  Divide1/1 -> Add2/1, Add1/2, Relational Operator/2
  Reference/1 -> Add1/1, Add2/2, Abs1/1, Add/2
  Signal/1 -> Data Type Conversion3/1, Add/1
  Add/1 -> Abs/1
  Abs/1 -> Relational Operator/1

== system Pedal_Interpretation_exe_gr/Test Specification for PI/SR-PI-02.2 Acceleration pedal interpretation/T_des_Drive increases/Detect increase ==
  Signal : Inport  OutDataType=sfix(16)  OutScaling=2^0
  Clock : Clock
      settings: Decimation=10
  Memory : Memory
  Relational Operator : RelationalOperator  LogicOutDataTypeMode=Specify via dialog
  Switch : Switch  Criteria=u2 > Threshold
  Increase : Outport  OutDataType=sfix(16)  OutScaling=2^0
  wires:
  Signal/1 -> Relational Operator/1, Memory/1, Switch/3
  Relational Operator/1 -> Increase/1
  Clock/1 -> Switch/2
  Memory/1 -> Switch/1
  Switch/1 -> Relational Operator/2
